simulink model "vehicle_brakes"  (R2022a)
settings: Solver=ode23t  StartTime=0.0  StopTime=75  RelTol=1e-3  AbsTol=1e-3  EnableMultiTasking=on
InitFcn:
  | load('terrain_data.mat');
  | car_tire_data;
undefined symbols (not defined in the file): rider_mass, tire_dia, vehicle_mass
libraries: fl_lib x7, nesl_utility x7, sdl_lib x5, fl_ps_legacy_lib x1
settings Model: Creator=sseshadr  LastModifiedBy=Andrew
settings SolverCC: AutoScaleAbsTol=off  AlgebraicLoopSolver=TrustRegion
settings DataIOCC: LimitDataPoints=on  SaveFormat=Array  ReturnWorkspaceOutputs=off
settings OptimizationCC: LifeSpan=inf
settings DebuggingCC: UnconnectedInputMsg=warning  UnconnectedOutputMsg=warning  UnconnectedLineMsg=warning  SFUnexpectedBacktrackingDiag=warning  SFNoUnconditionalDefaultTransitionDiag=warning  SFExecutionAtInitializationDiag=none  SFMachineParentedDataDiag=warning  ArithmeticOperatorsInVariantConditions=warning
settings HardwareCC: ProdBitPerPointer=32  ProdBitPerSizeT=32  ProdBitPerPtrDiffT=32  ProdLargestAtomicFloat=None  ProdIntDivRoundTo=Undefined  ProdEndianess=Unspecified  ProdWordSize=32  ProdHWDeviceType=32-bit Generic
settings ModelReferenceCC: PropagateSignalLabelsOutOfModel=off
settings SFSimCC: SimUseLocalCustomCode=off  CustomCodeUndefinedFunction=UseInterfaceOnly
settings RTWCC: RTWUseLocalCustomCode=off
settings CodeAppCC: StateflowObjectComments=on
settings GRTTargetCC: TargetLangStandard=C89/C90 (ANSI)
settings ConfigComp: CovMetricSettings=dw  CovSaveCumulativeToWorkspaceVar=on  CovSaveSingleToWorkspaceVar=on  CovExternalEMLEnable=off
settings SimscapeCC: SimscapeNormalizeSystem=off  SimscapeLogType=all  SimscapeLogDataHistory=10000

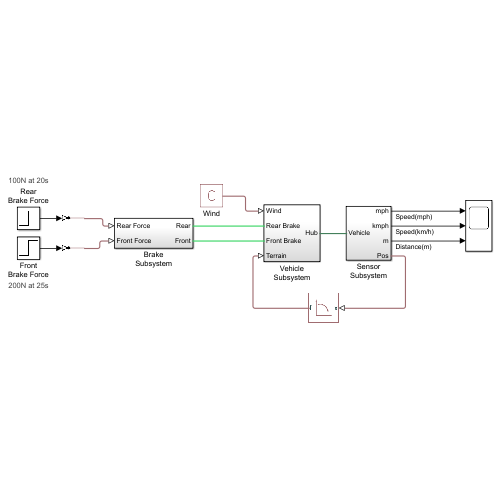
[thumbnail: Simulink's stored preview of the top-level diagram]
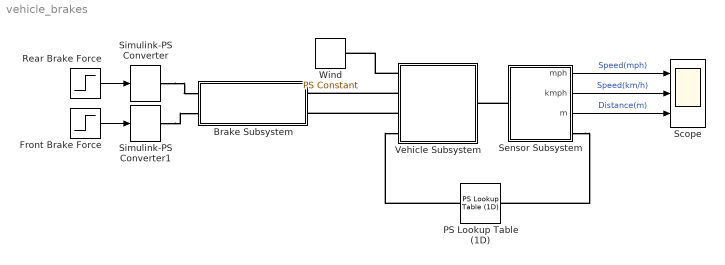
== system vehicle_brakes ==
  Brake Subsystem : Subsystem
  Front Brake Force : Step  Time=25  After=200  SampleTime=0
      settings: AttributesFormatString=%<After>N at %<Time>s
  PS Lookup Table (1D) : fl_ps_legacy_lib/Legacy Physical Signals/Lookup Tables/PS Lookup Table (1D)  x=dist  f=slope  interp_method=1  extrap_method=1
      settings: SourceProductBaseCode=PW,SS,VE  InternalSimscapePortConfiguration="{\"Bottom\":[],\"Left\":[{\"id\":\"I\",\"label\":\"x\",\"type\":\"input\"}],\"Right\":[{\"id\":\"O\",\"label\":\"f\",\"type\":\"output\"}],\"Top\":[]}"
  Rear Brake Force : Step  Time=20  After=100  SampleTime=0
      settings: AttributesFormatString=%<After>N at %<Time>s
  Scope : Scope  NumInputPorts=3
  Sensor Subsystem : Subsystem
  Simulink-PS Converter : nesl_utility/Simulink-PS Converter  PhysicalDomain=network_engine_domain  SubClassName=ps_input  LeftPortType=input  RightPortType=output  PseudoPeriodic=off  Frequencies=[]  NoiseDistribution=none  NoiseParameters=[]  Unit=1  AffineConversion=off  FilteringAndDerivatives=filter  SimscapeFilterOrder=1  InputFilterTimeConstant=0.001  UdotUserProvided=1
      settings: SourceProductBaseCode=SS,PW,VE
  Simulink-PS Converter1 : nesl_utility/Simulink-PS Converter  PhysicalDomain=network_engine_domain  SubClassName=ps_input  LeftPortType=input  RightPortType=output  PseudoPeriodic=off  Frequencies=[]  NoiseDistribution=none  NoiseParameters=[]  Unit=1  AffineConversion=off  FilteringAndDerivatives=filter  SimscapeFilterOrder=1  InputFilterTimeConstant=0.001  UdotUserProvided=1
      settings: SourceProductBaseCode=SS,PW,VE
  Vehicle Subsystem : Subsystem
  Wind : fl_lib/Physical Signals/Sources/PS Constant  constant=0
      settings: SourceProductBaseCode=PW,SS,VE
  wires:
  Sensor Subsystem/1(mph) -> Scope/1  "Speed(mph)"
  Sensor Subsystem/2(kmph) -> Scope/2  "Speed(km/h)"
  Sensor Subsystem/3(m) -> Scope/3  "Distance(m)"
  Rear Brake Force/1 -> Simulink-PS Converter/1
  Front Brake Force/1 -> Simulink-PS Converter1/1
  connections:
  Sensor Subsystem/LConn1 -- Vehicle Subsystem/RConn1
  Sensor Subsystem/RConn1 -- PS Lookup Table (1D)/LConn1
  PS Lookup Table (1D)/RConn1 -- Vehicle Subsystem/LConn4
  Simulink-PS Converter/RConn1 -- Brake Subsystem/LConn1
  Vehicle Subsystem/LConn2 -- Brake Subsystem/RConn1
  Vehicle Subsystem/LConn3 -- Brake Subsystem/RConn2
  Simulink-PS Converter1/RConn1 -- Brake Subsystem/LConn2
  Vehicle Subsystem/LConn1 -- Wind/RConn1

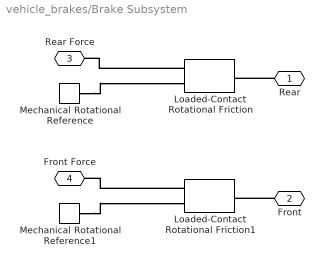
== system vehicle_brakes/Brake Subsystem ==
  Loaded-Contact Rotational Friction : sdl_lib/Brakes & Detents/Rotational/Loaded-Contact Rotational Friction  geometry_model=1  r_eff=280 mm  d_o=150 mm  d_i=100 mm  friction_model=1  mu_w_vector=[ 0 0.1 0.2 0.3 0.4 0.5 1 2 5 10 100 1000 ] rad/s  temperature_TLU=[280, 300, 320] K  mu_static=0.35  mu_static_vector=[.4, .38, .36]  mu_coulomb=0.3  mu_coulomb_vector=[ 0.29 0.28 0.26 0.22 0.21 0.2 0.2 0.19 0.19 0.19 0.19 0.19 ]  mu_coulomb_temp_vector=[.3, .28, .25]  mu_coulomb_matrix=[.34, .32, .3; .3, .28, .25; .25, .2, .15]  mu_interp_method=1  mu_extrap_method=1  w_tol=0.001 rad/s  force_min=1 N  mu_visc=0 N*m/(rad/s)  initial_state_locked=0  enable_faults=simscape.enum.onoff.off  fault_type=sdl.enum.clutchFault.lock  external_fault=simscape.enum.onoff.off  temporal_fault=simscape.enum.onoff.off  fault_time=5 s  report_fault=simscape.enum.assert.action.none  thermal_mass=50 kJ/K  T_init=300 K
      settings: SourceProductBaseCode=LD  InternalSimscapePortConfiguration="{\"Bottom\":[],\"Left\":[{\"id\":\"N\",\"label\":\"N\",\"type\":\"input\"},{\"id\":\"B\",\"label\":\"B\",\"type\":\"foundation.mechanical.rotational.rotational\"}],\"Right\":[{\"id\":\"F\",\"label\":\"F\",\"type\":\"foundation.mechanical.rotational.rotational\"}],\"Top\":[]}"
  Loaded-Contact Rotational Friction1 : sdl_lib/Brakes & Detents/Rotational/Loaded-Contact Rotational Friction  geometry_model=1  r_eff=280 mm  d_o=150 mm  d_i=100 mm  friction_model=1  mu_w_vector=[ 0 0.1 0.2 0.3 0.4 0.5 1 2 5 10 100 1000 ] rad/s  temperature_TLU=[280, 300, 320] K  mu_static=0.35  mu_static_vector=[.4, .38, .36]  mu_coulomb=0.3  mu_coulomb_vector=[ 0.29 0.28 0.26 0.22 0.21 0.2 0.2 0.19 0.19 0.19 0.19 0.19 ]  mu_coulomb_temp_vector=[.3, .28, .25]  mu_coulomb_matrix=[.34, .32, .3; .3, .28, .25; .25, .2, .15]  mu_interp_method=1  mu_extrap_method=1  w_tol=0.001 rad/s  force_min=1 N  mu_visc=0 N*m/(rad/s)  initial_state_locked=0  enable_faults=simscape.enum.onoff.off  fault_type=sdl.enum.clutchFault.lock  external_fault=simscape.enum.onoff.off  temporal_fault=simscape.enum.onoff.off  fault_time=5 s  report_fault=simscape.enum.assert.action.none  thermal_mass=50 kJ/K  T_init=300 K
      settings: SourceProductBaseCode=LD  InternalSimscapePortConfiguration="{\"Bottom\":[],\"Left\":[{\"id\":\"N\",\"label\":\"N\",\"type\":\"input\"},{\"id\":\"B\",\"label\":\"B\",\"type\":\"foundation.mechanical.rotational.rotational\"}],\"Right\":[{\"id\":\"F\",\"label\":\"F\",\"type\":\"foundation.mechanical.rotational.rotational\"}],\"Top\":[]}"
  Mechanical Rotational Reference : fl_lib/Mechanical/Rotational Elements/Mechanical Rotational Reference
      settings: SourceProductBaseCode=PW,SS,VE
  Mechanical Rotational Reference1 : fl_lib/Mechanical/Rotational Elements/Mechanical Rotational Reference
      settings: SourceProductBaseCode=PW,SS,VE
  Rear : PMIOPort  Side=Right
  Front : PMIOPort  Port=2  Side=Right
  Rear Force : PMIOPort  Port=3  Side=Left
  Front Force : PMIOPort  Port=4  Side=Left
  connections:
  Mechanical Rotational Reference/LConn1 -- Loaded-Contact Rotational Friction/LConn2
  Mechanical Rotational Reference1/LConn1 -- Loaded-Contact Rotational Friction1/LConn2
  Loaded-Contact Rotational Friction/LConn1 -- Rear Force/RConn1
  Loaded-Contact Rotational Friction1/LConn1 -- Front Force/RConn1
  Rear/RConn1 -- Loaded-Contact Rotational Friction/RConn1
  Front/RConn1 -- Loaded-Contact Rotational Friction1/RConn1

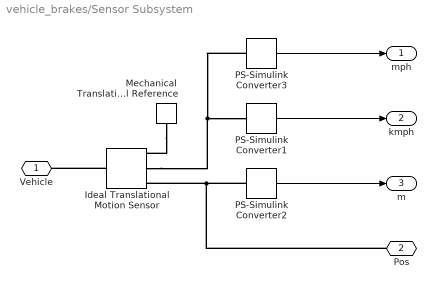
== system vehicle_brakes/Sensor Subsystem ==
  Ideal Translational Motion Sensor : fl_lib/Mechanical/Mechanical Sensors/Ideal Translational Motion Sensor  offset=0 m
      settings: SourceProductBaseCode=PW,SS,VE
  Mechanical Translational Reference : fl_lib/Mechanical/Translational Elements/Mechanical Translational Reference
      settings: SourceProductBaseCode=PW,SS,VE
  PS-Simulink Converter1 : nesl_utility/PS-Simulink Converter  PhysicalDomain=network_engine_domain  SubClassName=ps_output  LeftPortType=input  RightPortType=output  PseudoPeriodic=off  Frequencies=[]  VectorFormat=1-D array  Unit=km/hr  AffineConversion=off
      settings: SourceProductBaseCode=SS,PW,VE
  PS-Simulink Converter2 : nesl_utility/PS-Simulink Converter  PhysicalDomain=network_engine_domain  SubClassName=ps_output  LeftPortType=input  RightPortType=output  PseudoPeriodic=off  Frequencies=[]  VectorFormat=1-D array  Unit=1  AffineConversion=off
      settings: SourceProductBaseCode=SS,PW,VE
  PS-Simulink Converter3 : nesl_utility/PS-Simulink Converter  PhysicalDomain=network_engine_domain  SubClassName=ps_output  LeftPortType=input  RightPortType=output  PseudoPeriodic=off  Frequencies=[]  VectorFormat=1-D array  Unit=mph  AffineConversion=off
      settings: SourceProductBaseCode=SS,PW,VE
  Vehicle : PMIOPort  Side=Left
  Pos : PMIOPort  Port=2  Side=Right
  mph : Outport  VectorParamsAs1DForOutWhenUnconnected=off
  kmph : Outport  Port=2  VectorParamsAs1DForOutWhenUnconnected=off
  m : Outport  Port=3  VectorParamsAs1DForOutWhenUnconnected=off
  wires:
  PS-Simulink Converter1/1 -> kmph/1
  PS-Simulink Converter2/1 -> m/1
  PS-Simulink Converter3/1 -> mph/1
  connections:
  Mechanical Translational Reference/LConn1 -- Ideal Translational Motion Sensor/RConn1
  PS-Simulink Converter2/LConn1 -- Pos/RConn1 -- Ideal Translational Motion Sensor/RConn3
  Ideal Translational Motion Sensor/RConn2 -- PS-Simulink Converter3/LConn1 -- PS-Simulink Converter1/LConn1
  Ideal Translational Motion Sensor/LConn1 -- Vehicle/RConn1

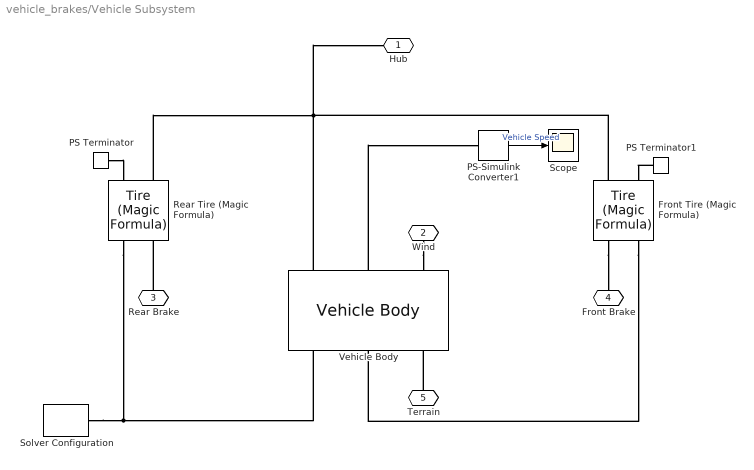
== system vehicle_brakes/Vehicle Subsystem ==
  Front Tire (Magic Formula) : sdl_lib/Tires & Vehicles/Tire (Magic Formula)  parameterization=2  F_z1=3e+3 N  F_x1=3.5e+3 N  kappa1=10  B_m=tire_b  C_m=tire_c  D_m=tire_d  E_m=tire_e  fz0=4e+3 N  p_Cx=1.685  p_Dx=[ 1.21 -0.037 ]  p_Ex=[ 0.344 0.095 -0.02 0 ]  p_Kx=[ 21.51 -0.163 0.245 ]  p_Hx=[ -0.002 0.002 ]  p_Vx=[ 0 0 ]  r_e=tire_dia/2 in  model_compliance=0  stiffness=1e+6 N/m  damping=1000 N/(m/s)  model_inertia=1  inertia=tire_inertia kg*m^2  initial_velocity=0 rad/s  model_resistance=1  resistance_model=1  coeff=roll_resist  p_tire=250e3 Pa  alpha=-0.003  beta=0.97  coeff_a=84e-4  coeff_b=6.2e-4 s/m  coeff_c=1.6e-4 s^2/m^2  v_thr=1e-3 m/s  v_tr_thr=0.1 m/s
  PS Terminator : fl_lib/Physical Signals/Sinks/PS Terminator
      settings: SourceProductBaseCode=PW,SS,VE
  PS Terminator1 : fl_lib/Physical Signals/Sinks/PS Terminator
      settings: SourceProductBaseCode=PW,SS,VE
  PS-Simulink Converter1 : nesl_utility/PS-Simulink Converter  PhysicalDomain=network_engine_domain  SubClassName=ps_output  LeftPortType=input  RightPortType=output  PseudoPeriodic=off  Frequencies=[]  VectorFormat=1-D array  Unit=1  AffineConversion=off
      settings: SourceProductBaseCode=SS,PW,VE
  Rear Tire (Magic Formula) : sdl_lib/Tires & Vehicles/Tire (Magic Formula)  parameterization=2  F_z1=3e+3 N  F_x1=3.5e+3 N  kappa1=10  B_m=tire_b  C_m=tire_c  D_m=tire_d  E_m=tire_e  fz0=4e+3 N  p_Cx=1.685  p_Dx=[ 1.21 -0.037 ]  p_Ex=[ 0.344 0.095 -0.02 0 ]  p_Kx=[ 21.51 -0.163 0.245 ]  p_Hx=[ -0.002 0.002 ]  p_Vx=[ 0 0 ]  r_e=tire_dia/2 in  model_compliance=0  stiffness=1e+6 N/m  damping=1000 N/(m/s)  model_inertia=1  inertia=tire_inertia kg*m^2  initial_velocity=0 rad/s  model_resistance=1  resistance_model=1  coeff=roll_resist  p_tire=250e3 Pa  alpha=-0.003  beta=0.97  coeff_a=84e-4  coeff_b=6.2e-4 s/m  coeff_c=1.6e-4 s^2/m^2  v_thr=1e-3 m/s  v_tr_thr=0.1 m/s
  Scope : Scope
  Solver Configuration : nesl_utility/Solver Configuration  PhysicalDomain=network_engine_domain  SubClassName=solver  LeftPortType=input  RightPortType=generic  Tones=[]  Harmonics=[]  SimulateNoise=off  Profile=off  UseLocalSampling=off  EnableSwitchedLinearOptims=on  FrequencyDomain=off  UseCCode=off  RelTol=0.001  AbsTol=1e-06  MinStep=1e-09  ToWorkspace=off  RevertToSquareIcSolve=off  NumHomotopyIterations=100  PhasorMode=off  PhasorModeNumHarmonics=1  IndexReductionMethod=DerivativeReplacement  DoDC=off  ResidualTolerance=1e-09  UseLocalSolver=off  LocalSolverChoice=NE_BACKWARD_EULER_ADVANCER  LocalSolverSampleTime=0.001  DoFixedCost=off  MaxNonlinIter=3  MaxModeIter=2  ComputeImpulses=off  ImpulseIterations=2  LinearAlgebra=Sparse  LinearAlgebraNumThread=0  EquationFormulation=NE_TIME_EF  DelaysMemoryBudget=1024  AutomaticFiltering=on  FilteringTimeConstant=0.001  PartitionStorageMethod=AS_NEEDED  PartitionMemoryBudget=1024  PartitionMethod=FAST
      settings: SourceProductBaseCode=SS,PW,VE
  Vehicle Body : sdl_lib/Tires & Vehicles/Vehicle Body  mass=rider_mass + vehicle_mass kg  n_w=1  x_f=front_axle mm  x_r=rear_axle mm  y_c=CG_height mm  mass_var=simscape.enum.onoff.off  g=9.81 m/s^2  liftoff_warning=simscape.enum.onoff.off  area=front_area m^2  Cd=drag_coeff  rho=1.18 kg/m^3  model_pitch=simscape.enum.onoff.off  inertia=4000 kg*m^2  suspension_model=sdl.enum.linearTLU.linear  k_f=1e4 N/m  b_f=1e4 N*s/m  k_r=1e4 N/m  b_r=1e4 N*s/m  k_f_TLU=[-2000, -1000, 0, 1000, 2000] N  x_f_TLU=[-.4, -.2, 0, .2, .4] m  b_f_TLU=[-200, -100, 0, 100, 200] N  v_f_TLU=[-4, -2, 0, 2, 4] m/s  k_r_TLU=[-2000, -1000, 0, 1000, 2000] N  x_r_TLU=[-.4, -.2, 0, .2, .4] m  b_r_TLU=[-200, -100, 0, 100, 200] N  v_r_TLU=[-4, -2, 0, 2, 4] m/s  interp_method=simscape.enum.interpolation.linear  extrap_method=simscape.enum.extrapolation.linear  model_hardstop=simscape.enum.onoff.off  upper_bound_f=.25 m  lower_bound_f=-.25 m  stop_k_f=1e6 N/m  stop_b_f=150 N*s/m  upper_bound_r=.25 m  lower_bound_r=-.25 m  stop_k_r=1e6 N/m  stop_b_r=150 N*s/m  initial_pitch=0 rad  initial_pitch_rate=0 rad/s  v_specify=on  v_priority=High  v=0 m/s  v_nominal_specify=off  v_nominal_unit=m/s  v_nominal_value=1
  Hub : PMIOPort  Side=Right
  Wind : PMIOPort  Port=2  Side=Left
  Rear Brake : PMIOPort  Port=3  Side=Left
  Front Brake : PMIOPort  Port=4  Side=Left
  Terrain : PMIOPort  Port=5  Side=Left
  wires:
  PS-Simulink Converter1/1 -> Scope/1  "Vehicle Speed"
  connections:
  Rear Tire (Magic Formula)/LConn1 -- Solver Configuration/RConn1 -- Vehicle Body/RConn1
  Front Tire (Magic Formula)/RConn2 -- Hub/RConn1 -- Rear Tire (Magic Formula)/RConn2 -- Vehicle Body/LConn1
  Vehicle Body/LConn2 -- PS-Simulink Converter1/LConn1
  Front Tire (Magic Formula)/LConn1 -- Vehicle Body/RConn2
  Rear Brake/RConn1 -- Rear Tire (Magic Formula)/LConn2
  PS Terminator1/LConn1 -- Front Tire (Magic Formula)/RConn1
  PS Terminator/LConn1 -- Rear Tire (Magic Formula)/RConn1
  Front Tire (Magic Formula)/LConn2 -- Front Brake/RConn1
  Wind/RConn1 -- Vehicle Body/LConn3
  Terrain/RConn1 -- Vehicle Body/RConn3
